simulink model "Regulation_Case"  (R2021a)
settings: Solver=VariableStepAuto  StartTime=0.0  StopTime=600  RelTol=1e-3
values from neighbouring files (symbols this model uses):
  kd = 150    [Parameters.m]
  kp = 10    [Parameters.m]
  omega0 = [0.01 0.01 0.01]'    [Parameters.m]
  q0 = (1/sqrt(2))*[1 0 0 1]'    [Parameters.m]
  qc = [0 0 0 1]'    [Parameters.m]
settings Model: Creator=VTX  LastModifiedBy=VTX

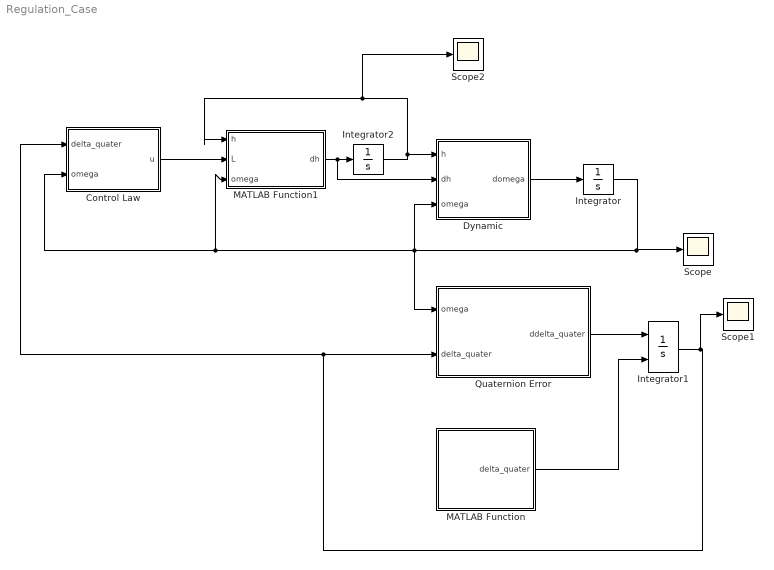
== system Regulation_Case ==
  Control Law : MATLAB Function  TreatAsAtomicUnit=on
  Dynamic : MATLAB Function  TreatAsAtomicUnit=on
  Integrator : Integrator  InitialCondition=omega0
  Integrator1 : Integrator  InitialConditionSource=external
  Integrator2 : Integrator  InitialCondition=[0 0 0]'
  MATLAB Function : MATLAB Function  TreatAsAtomicUnit=on
  MATLAB Function1 : MATLAB Function  TreatAsAtomicUnit=on
  Quaternion Error : MATLAB Function  TreatAsAtomicUnit=on
  Scope : Scope
  Scope1 : Scope
  Scope2 : Scope
  wires:
  Dynamic/1(domega) -> Integrator/1
  Quaternion Error/1(ddelta_quater) -> Integrator1/1
  MATLAB Function/1(delta_quater) -> Integrator1/2
  Integrator1/1 -> Scope1/1, Control Law/1(delta_quater), Quaternion Error/2(delta_quater)
  Integrator/1 -> Scope/1, MATLAB Function1/3(omega), Control Law/2(omega), Quaternion Error/1(omega), Dynamic/3(omega)
  Control Law/1(u) -> MATLAB Function1/2(L)
  MATLAB Function1/1(dh) -> Dynamic/2(dh), Integrator2/1
  Integrator2/1 -> Dynamic/1(h), Scope2/1, MATLAB Function1/1(h)

== matlab function Regulation_Case/MATLAB Function ==
  data: delta_quater output; q0 parameter; qc parameter
function delta_quater = fcn(q0, qc)
    delta_quater_1to3 = property_matrix(qc)'*q0;
    delta_quater4 = q0'*qc;
    
    delta_quater = [delta_quater_1to3' delta_quater4]';
end

== matlab function Regulation_Case/Dynamic ==
  data: h input; dh input; domega output; omega input; J parameter
function domega = fcn(h,dh,omega, J)
    domega = -inv(J)*(cross_matrix(omega)*(J*omega + h) + dh);
end

== matlab function Regulation_Case/Control Law ==
  data: delta_quater input; u output; omega input; kp parameter; kd parameter
function u = fcn(delta_quater,omega, kp, kd)
    %u = -kp*delta_quater(1:3) - kd*(1 + delta_quater(1:3)'*delta_quater(1:3))*omega;
    u = -kp*sign(delta_quater(4))*delta_quater(1:3) - kd*omega;
end

== matlab function Regulation_Case/Quaternion Error ==
  data: ddelta_quater output; omega input; delta_quater input
function ddelta_quater = fcn(omega, delta_quater)
    ddelta_quater_1to3 = (cross_matrix(delta_quater(1:3))*omega + delta_quater(4)*omega)/2;
    ddelta_quater4 = -0.5*delta_quater(1:3)'*omega;
    
    ddelta_quater = [ddelta_quater_1to3' ddelta_quater4]';
end

== matlab function Regulation_Case/MATLAB Function1 ==
  data: dh output; h input; L input; omega input
function dh = fcn(h, L, omega)
    dh = -cross_matrix(omega)*h - L;
end
